simulink model "UltraSonic_Sensor"  (R2020b)
settings: Solver=FixedStepDiscrete  StartTime=0.0  StopTime=10  FixedStep=1e-4  MaxStep=0.1  RelTol=1e-3
settings Model: DataDictionary=pid.sldd  Creator=The MathWorks, Inc.  LastModifiedBy=moody
settings DataIOCC: SaveFormat=Array  SaveOutput=off  SaveTime=off
settings OptimizationCC: DefaultParameterBehavior=Inlined  UseDivisionForNetSlopeComputation=on  GainParamInheritBuiltInType=on  UseFloatMulNetSlope=on  InlineInvariantSignals=on  ExpressionDepthLimit=2147483647  NoFixptDivByZeroProtection=on  EfficientFloat2IntCast=on  LifeSpan=1  OptimizeBlockOrder=speed  DifferentSizesBufferReuse=on  EfficientTunableParamExpr=on
settings DebuggingCC: MergeDetectMultiDrivingBlocksExec=none  SolverPrmCheckMsg=warning  ParameterTunabilityLossMsg=error  AllowSymbolicDim=off  ModelReferenceSymbolNameMessage=none  StateNameClashWarn=warning  SFUnexpectedBacktrackingDiag=warning  SFNoUnconditionalDefaultTransitionDiag=warning  SFExecutionAtInitializationDiag=none  ArithmeticOperatorsInVariantConditions=warning
settings HardwareCC: ProdBitPerPointer=32  ProdBitPerSizeT=32  ProdBitPerPtrDiffT=32  ProdLargestAtomicInteger=Long  ProdLargestAtomicFloat=Double  ProdWordSize=32  ProdHWDeviceType=ARM Compatible->ARM Cortex-M
settings ModelReferenceCC: PropagateSignalLabelsOutOfModel=off
settings SFSimCC: SimUseLocalCustomCode=off  MATLABDynamicMemAlloc=off  CustomCodeUndefinedFunction=UseInterfaceOnly
settings RTWCC: Description=Embedded Coder  SystemTargetFile=ert.tlc  GenCodeOnly=on  TemplateMakefile=ert_default_tmf  GenerateReport=on  RTWUseLocalCustomCode=off  LaunchReport=on
settings CodeAppCC: ForceParamTrailComments=on  IgnoreCustomStorageClasses=off  OperatorAnnotations=on  SimulinkDataObjDesc=on  SFDataObjDesc=on  CustomSymbolStrGlobalVar=rt$N$M  CustomSymbolStrType=$N$M  CustomSymbolStrFcn=$N$M$F  CustomSymbolStrMacro=$N$M  InsertBlockDesc=on
settings ERTTargetCC: GenerateSampleERTMain=on  CombineSignalStateStructs=on  SupportAbsoluteTime=off  CodeInterfacePackaging=Reusable function  SupportNonFinite=off  SupportComplex=off  SupportNonInlinedSFcns=on  InlinedParameterPlacement=NonHierarchical  RootIOFormat=Structure reference  ERTSrcFileBannerTemplate=code_c_template.cgt  ERTHdrFileBannerTemplate=code_h_template.cgt  ERTDataSrcFileTemplate=data_c_template.cgt  ERTDataHdrFileTemplate=data_h_template.cgt  ERTCustomFileTemplate=example_file_process.tlc  ERTFilePackagingFormat=Compact  EnableSignedLeftShifts=off
settings ConfigComp: CovMetricSettings=dw  CovSaveCumulativeToWorkspaceVar=on  CovSaveSingleToWorkspaceVar=on  CovExternalEMLEnable=off  CovSFcnEnable=off

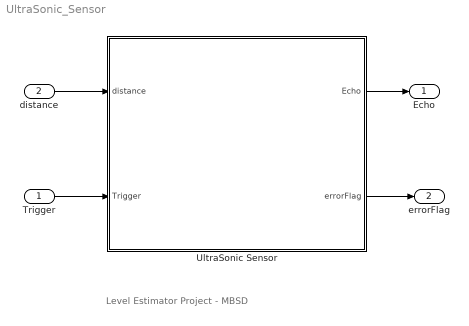
== system UltraSonic_Sensor ==
  note: Level Estimator Project - MBSD
  Trigger : Inport  OutDataTypeStr=boolean  PortDimensions=1
  distance : Inport  Port=2  OutDataTypeStr=uint16  PortDimensions=1
  UltraSonic Sensor : Subsystem
      mask Display: image('$imagefile'); % Use "Edit Image" on toolstrip to change.
  Echo : Outport  OutDataTypeStr=boolean  PortDimensions=1
  errorFlag : Outport  Port=2  OutDataTypeStr=boolean  PortDimensions=1
  wires:
  UltraSonic Sensor/1(Echo) -> Echo/1
  UltraSonic Sensor/2(errorFlag) -> errorFlag/1
  distance/1 -> UltraSonic Sensor/1(distance)
  Trigger/1 -> UltraSonic Sensor/2(Trigger)

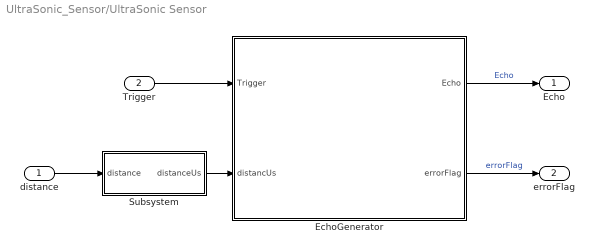
== system UltraSonic_Sensor/UltraSonic Sensor ==
  distance : Inport  OutDataTypeStr=uint16  PortDimensions=1
  Trigger : Inport  Port=2  OutDataTypeStr=boolean  PortDimensions=1
  EchoGenerator : Stateflow chart  TreatAsAtomicUnit=on
  Subsystem : Subsystem
  Echo : Outport  OutDataTypeStr=boolean  PortDimensions=1
  errorFlag : Outport  Port=2  OutDataTypeStr=boolean  PortDimensions=1
  wires:
  distance/1 -> Subsystem/1(distance)
  EchoGenerator/2(errorFlag) -> errorFlag/1  "errorFlag"
  Subsystem/1(distanceUs) -> EchoGenerator/2(distancUs)
  EchoGenerator/1(Echo) -> Echo/1  "Echo"
  Trigger/1 -> EchoGenerator/1(Trigger)

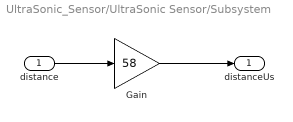
== system UltraSonic_Sensor/UltraSonic Sensor/Subsystem ==
  distance : Inport  OutDataTypeStr=uint16  PortDimensions=1
  Gain : Gain  Gain=58  OutDataTypeStr=uint16
  distanceUs : Outport  OutDataTypeStr=uint16  PortDimensions=1
  wires:
  distance/1 -> Gain/1
  Gain/1 -> distanceUs/1

== stateflow chart UltraSonic_Sensor/UltraSonic Sensor/EchoGenerator ==
  state watingTriggerHigh
    entry:
    Echo = false;
    errorFlag = false;
  state calculateTriggetDuration
    entry, during, exit:
    triggerDuraion = elapsed(msec);
  state flagError
    entry:
    errorFlag = true;
  state watingEchoLatency
    entry:
    Echo = false;
  state echoOn
    entry:
    Echo = true;
  state echoOff
    entry:
    Echo = false;
  (default) -> watingTriggerHigh
  (junction 136) -> watingTriggerHigh
  flagError -> (junction 136) : after(100, msec)
  (junction 253) -> watingTriggerHigh
  watingTriggerHigh -> calculateTriggetDuration : [Trigger == true]
  calculateTriggetDuration -> flagError [order 2] : [Trigger == false && triggerDuraion < 9]
  calculateTriggetDuration -> watingEchoLatency [order 1] : [Trigger == false && triggerDuraion >= 9]
  watingEchoLatency -> (junction 253) [order 2] : [distancUs == 0]
  echoOff -> (junction 253)
  watingEchoLatency -> echoOn [order 1] : after(2, msec)[distancUs ~= 0]
  echoOn -> echoOff : after(distancUs, usec)
  data: Trigger input boolean size=1; triggerDuraion local double size=1 =0; Echo output boolean size=1; errorFlag output boolean size=1; distancUs input uint16 size=1
